simulink model "Invertedpendulumsim"  (R2021a)
settings: Solver=VariableStepAuto  StartTime=0.0  StopTime=10.0  MaxStep=0.01  MinStep=0.001  RelTol=1e-6
values from neighbouring files (symbols this model uses):
  A = [0 1 0 0;8.175 0 0 0; 0 0 0 1; -3.27 0 0 0]    [Inverted_pend_script.m]
  B = [0;-0.33; 0; 0.467]    [Inverted_pend_script.m]
  C = [1 0 0 0; 0 1 0 0;0 0 1 0;0 0 0 1]    [Inverted_pend_script.m]
  D = [0;0;0;0]    [Inverted_pend_script.m]
  K = acker(A,B,[-4+2i -4-2i -10 -10])    [Inverted_pend_script.m]
settings Model: Creator=siddi  LastModifiedBy=siddi

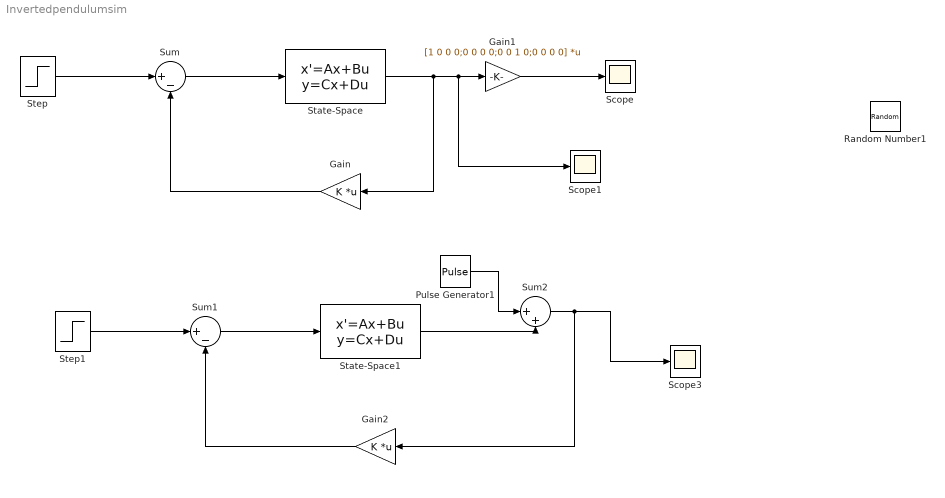
== system Invertedpendulumsim ==
  Gain : Gain  Gain=K  Multiplication=Matrix(K*u)
  Gain1 : Gain  Gain=[1 0 0 0;0 0 0 0;0 0 1 0;0 0 0 0]  Multiplication=Matrix(K*u)
  Gain2 : Gain  Gain=K  Multiplication=Matrix(K*u)
  Pulse Generator1 : DiscretePulseGenerator  PulseType=Time based  Period=10  PulseWidth=5
  Random Number1 : RandomNumber  SampleTime=0.1
  Scope : Scope
  Scope1 : Scope
  Scope3 : Scope
  State-Space : StateSpace  A=A  B=B  C=C  D=D  InitialCondition=[2 2 0 0];
  State-Space1 : StateSpace  A=A  B=B  C=C  D=D  InitialCondition=[2 2 0 0];
  Step : Step  SampleTime=0
  Step1 : Step  After=2  SampleTime=0
  Sum : Sum  Inputs=|+-
  Sum1 : Sum  Inputs=|+-
  Sum2 : Sum  Inputs=|++
  wires:
  Step/1 -> Sum/1
  Sum/1 -> State-Space/1
  State-Space/1 -> Gain/1, Scope1/1, Gain1/1
  Gain1/1 -> Scope/1
  Gain/1 -> Sum/2
  Step1/1 -> Sum1/1
  Gain2/1 -> Sum1/2
  Sum1/1 -> State-Space1/1
  State-Space1/1 -> Sum2/2
  Sum2/1 -> Gain2/1, Scope3/1
  Pulse Generator1/1 -> Sum2/1
